simulink subsystem "cvrs_ventricle_volume_diastole"  (R2019b)
settings: Solver=VariableStepAuto  StartTime=0.0  StopTime=10.0  RelTol=1e-3
undefined symbols (not defined in the file): __PRM__SERIALIZED__DATA__, SubsystemReferenceBlock
settings Model: Creator=RH  LastModifiedBy=RH

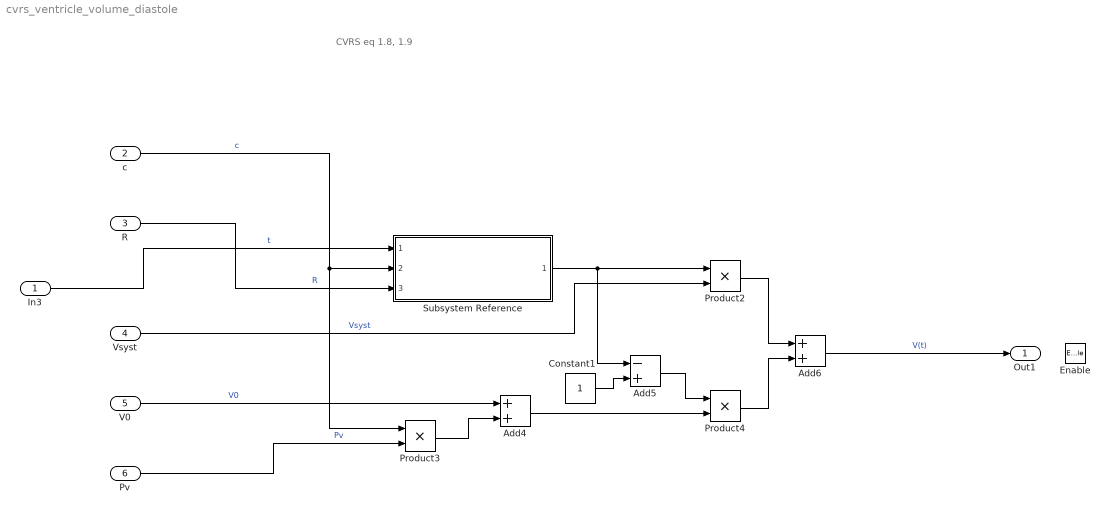
== system cvrs_ventricle_volume_diastole ==
  note: CVRS eq 1.8, 1.9
  In3 : Inport
  c : Inport  Port=2
  R : Inport  Port=3
  Vsyst : Inport  Port=4
  V0 : Inport  Port=5
  Pv : Inport  Port=6
  Enable : EnablePort
  Add4 : Sum
  Add5 : Sum  Inputs=-+
  Add6 : Sum
  Constant1 : Constant
  Product2 : Product
  Product3 : Product
  Product4 : Product
  Subsystem Reference : Subsystem  BlockKeywords=__PRM__SERIALIZED__DATA__:SubsystemReferenceBlock  ReferencedSubsystem=heart_cycle
  Out1 : Outport
  wires:
  Subsystem Reference/1 -> Product2/1, Add5/1
  c/1 -> Product3/1, Subsystem Reference/2  "c"
  Product2/1 -> Add6/1
  Product4/1 -> Add6/2
  Product3/1 -> Add4/2
  Vsyst/1 -> Product2/2  "Vsyst"
  Add4/1 -> Product4/2
  Constant1/1 -> Add5/2
  V0/1 -> Add4/1  "V0"
  Add5/1 -> Product4/1
  Pv/1 -> Product3/2  "Pv"
  Add6/1 -> Out1/1  "V(t)"
  R/1 -> Subsystem Reference/3  "R"
  In3/1 -> Subsystem Reference/1  "t"
